simulink model "case3"  (R2024b)
settings: Solver=FixedStepAuto  StartTime=0  StopTime=1  FixedStep=1e-7  RelTol=1e-3
values from neighbouring files (symbols this model uses):
  SG_D_1_D = 0.01056    [IEEE9_case_parameters.m]    (also in case1_parameters.m; case2_parameters.m; case3_parameters.m; case4_parameters.m)
  SG_D_1_EnableSaturation = 0    [IEEE9_case_parameters.m]    (also in case1_parameters.m; case2_parameters.m; case3_parameters.m; case4_parameters.m)
  SG_D_1_f0 = 60    [IEEE9_case_parameters.m]    (also in case1_parameters.m; case2_parameters.m; case3_parameters.m; case4_parameters.m)
  SG_D_1_H = 7.5    [IEEE9_case_parameters.m]    (also in case1_parameters.m; case2_parameters.m; case3_parameters.m; case4_parameters.m)
  SG_D_1_K_A = 20    [IEEE9_case_parameters.m]    (also in case1_parameters.m; case2_parameters.m; case3_parameters.m; case4_parameters.m)
  SG_D_1_K_E = 1.000000e+1    (= 10)    [IEEE9_case_parameters.m]    (also in case1_parameters.m; case2_parameters.m; case3_parameters.m; case4_parameters.m)
  SG_D_1_K_F = 2.363    [IEEE9_case_parameters.m]    (also in case1_parameters.m; case2_parameters.m; case3_parameters.m; case4_parameters.m)
  SG_D_1_K_s = 0.5    [IEEE9_case_parameters.m]    (also in case1_parameters.m = 5; case2_parameters.m = 5; case3_parameters.m = 5; case4_parameters.m = 5)
  SG_D_1_R_a = 0.001088    [IEEE9_case_parameters.m]    (also in case1_parameters.m; case2_parameters.m; case3_parameters.m; case4_parameters.m)
  SG_D_1_S_A = 1    [IEEE9_case_parameters.m]    (also in case1_parameters.m; case2_parameters.m; case3_parameters.m; case4_parameters.m)
  SG_D_1_S_B = 0.103    [IEEE9_case_parameters.m]    (also in case1_parameters.m; case2_parameters.m; case3_parameters.m; case4_parameters.m)
  SG_D_1_S_N = 10.659857    [IEEE9_case_parameters.m]    (also in case1_parameters.m; case2_parameters.m; case3_parameters.m; case4_parameters.m)
  SG_D_1_SpeedPara = 200    [IEEE9_case_parameters.m]    (also in case1_parameters.m; case2_parameters.m; case3_parameters.m; case4_parameters.m)
  SG_D_1_T_0 = 0.720173    [IEEE9_case_parameters.m]    (also in case1_parameters.m = 0.755522; case2_parameters.m = 0.808931; case3_parameters.m = 0.869402; case4_parameters.m = 0.729316)
  SG_D_1_T_1 = 0.3    [IEEE9_case_parameters.m]    (also in case1_parameters.m; case2_parameters.m; case3_parameters.m; case4_parameters.m)
  SG_D_1_T_2 = 0.05    [IEEE9_case_parameters.m]    (also in case1_parameters.m; case2_parameters.m; case3_parameters.m; case4_parameters.m)
  SG_D_1_T_3 = 0.02    [IEEE9_case_parameters.m]    (also in case1_parameters.m; case2_parameters.m; case3_parameters.m; case4_parameters.m)
  SG_D_1_T_4 = 0.005    [IEEE9_case_parameters.m]    (also in case1_parameters.m; case2_parameters.m; case3_parameters.m; case4_parameters.m)
  SG_D_1_T_A = 0.02    [IEEE9_case_parameters.m]    (also in case1_parameters.m; case2_parameters.m; case3_parameters.m; case4_parameters.m)
  SG_D_1_T_dd = 8.000000e+0    (= 8)    [IEEE9_case_parameters.m]    (also in case1_parameters.m; case2_parameters.m; case3_parameters.m; case4_parameters.m)
  SG_D_1_T_ddd = 0.04    [IEEE9_case_parameters.m]    (also in case1_parameters.m; case2_parameters.m; case3_parameters.m; case4_parameters.m)
  SG_D_1_T_E = 0.314    [IEEE9_case_parameters.m]    (also in case1_parameters.m; case2_parameters.m; case3_parameters.m; case4_parameters.m)
  SG_D_1_T_F = 0.35    [IEEE9_case_parameters.m]    (also in case1_parameters.m; case2_parameters.m; case3_parameters.m; case4_parameters.m)
  SG_D_1_T_qd = 0.8    [IEEE9_case_parameters.m]    (also in case1_parameters.m; case2_parameters.m; case3_parameters.m; case4_parameters.m)
  SG_D_1_T_qdd = 0.02    [IEEE9_case_parameters.m]    (also in case1_parameters.m; case2_parameters.m; case3_parameters.m; case4_parameters.m)
  SG_D_1_T_speed = 0.1    [IEEE9_case_parameters.m]    (also in case1_parameters.m = 200; case2_parameters.m = 200; case3_parameters.m = 200; case4_parameters.m = 200)
  SG_D_1_T_w = 0.5    [IEEE9_case_parameters.m]    (also in case1_parameters.m; case2_parameters.m; case3_parameters.m; case4_parameters.m)
  SG_D_1_V_ref = 1.990276    [IEEE9_case_parameters.m]    (also in case1_parameters.m = 2.042296; case2_parameters.m = 2.051388; case3_parameters.m = 2.089584; case4_parameters.m = 2.01845)
  SG_D_1_w_ref = 376.991118    [IEEE9_case_parameters.m]    (also in case1_parameters.m; case2_parameters.m; case3_parameters.m; case4_parameters.m)
  SG_D_1_wb = 6.000000e+1    (= 60)    [IEEE9_case_parameters.m]    (also in case1_parameters.m; case2_parameters.m; case3_parameters.m; case4_parameters.m)
  SG_D_1_x_d = 1.9    [IEEE9_case_parameters.m]    (also in case1_parameters.m; case2_parameters.m; case3_parameters.m; case4_parameters.m)
  SG_D_1_x_dd = 0.302    [IEEE9_case_parameters.m]    (also in case1_parameters.m; case2_parameters.m; case3_parameters.m; case4_parameters.m)
  SG_D_1_x_ddd = 0.204    [IEEE9_case_parameters.m]    (also in case1_parameters.m; case2_parameters.m; case3_parameters.m; case4_parameters.m)
  SG_D_1_x_l = 0.05    [IEEE9_case_parameters.m]    (also in case1_parameters.m; case2_parameters.m; case3_parameters.m; case4_parameters.m)
  SG_D_1_x_q = 1.3    [IEEE9_case_parameters.m]    (also in case1_parameters.m; case2_parameters.m; case3_parameters.m; case4_parameters.m)
  SG_D_1_x_qd = 0.5    [IEEE9_case_parameters.m]    (also in case1_parameters.m; case2_parameters.m; case3_parameters.m; case4_parameters.m)
  SG_D_1_x_qdd = 0.3    [IEEE9_case_parameters.m]    (also in case1_parameters.m; case2_parameters.m; case3_parameters.m; case4_parameters.m)
  SG_D_2_D = 0.02    [IEEE9_case_parameters.m]    (also in case1_parameters.m; case2_parameters.m; case3_parameters.m; case4_parameters.m)
  SG_D_2_EnableSaturation = 0    [IEEE9_case_parameters.m]    (also in case1_parameters.m; case2_parameters.m; case3_parameters.m; case4_parameters.m)
  SG_D_2_f0 = 60    [IEEE9_case_parameters.m]    (also in case1_parameters.m; case2_parameters.m; case3_parameters.m; case4_parameters.m)
  SG_D_2_H = 8.000000e+0    (= 8)    [IEEE9_case_parameters.m]    (also in case1_parameters.m; case2_parameters.m; case3_parameters.m; case4_parameters.m)
  SG_D_2_K_A = 20    [IEEE9_case_parameters.m]    (also in case1_parameters.m; case2_parameters.m; case3_parameters.m; case4_parameters.m)
  SG_D_2_K_E = 1.000000e+1    (= 10)    [IEEE9_case_parameters.m]    (also in case1_parameters.m; case2_parameters.m; case3_parameters.m; case4_parameters.m)
  SG_D_2_K_F = 2.363    [IEEE9_case_parameters.m]    (also in case1_parameters.m; case2_parameters.m; case3_parameters.m; case4_parameters.m)
  SG_D_2_K_s = 0.5    [IEEE9_case_parameters.m]    (also in case1_parameters.m = 4; case2_parameters.m = 4; case3_parameters.m = 4; case4_parameters.m = 4)
  SG_D_2_R_a = 0.001088    [IEEE9_case_parameters.m]    (also in case1_parameters.m; case2_parameters.m; case3_parameters.m; case4_parameters.m)
  SG_D_2_S_A = 1    [IEEE9_case_parameters.m]    (also in case1_parameters.m; case2_parameters.m; case3_parameters.m; case4_parameters.m)
  SG_D_2_S_B = 0.103    [IEEE9_case_parameters.m]    (also in case1_parameters.m; case2_parameters.m; case3_parameters.m; case4_parameters.m)
  SG_D_2_S_N = 10.659857    [IEEE9_case_parameters.m]    (also in case1_parameters.m; case2_parameters.m; case3_parameters.m; case4_parameters.m)
  SG_D_2_SpeedPara = 200    [IEEE9_case_parameters.m]    (also in case1_parameters.m; case2_parameters.m; case3_parameters.m; case4_parameters.m)
  SG_D_2_T_0 = 1.632913    [IEEE9_case_parameters.m]    (also in case1_parameters.m = 1.632925; case2_parameters.m = 1.632915; case3_parameters.m = 1.632914; case4_parameters.m = 1.632927)
  SG_D_2_T_1 = 0.2    [IEEE9_case_parameters.m]    (also in case1_parameters.m; case2_parameters.m; case3_parameters.m; case4_parameters.m)
  SG_D_2_T_2 = 0.05    [IEEE9_case_parameters.m]    (also in case1_parameters.m; case2_parameters.m; case3_parameters.m; case4_parameters.m)
  SG_D_2_T_3 = 0.02    [IEEE9_case_parameters.m]    (also in case1_parameters.m; case2_parameters.m; case3_parameters.m; case4_parameters.m)
  SG_D_2_T_4 = 0.005    [IEEE9_case_parameters.m]    (also in case1_parameters.m; case2_parameters.m; case3_parameters.m; case4_parameters.m)
  SG_D_2_T_A = 0.02    [IEEE9_case_parameters.m]    (also in case1_parameters.m; case2_parameters.m; case3_parameters.m; case4_parameters.m)
  SG_D_2_T_dd = 7.9    [IEEE9_case_parameters.m]    (also in case1_parameters.m; case2_parameters.m; case3_parameters.m; case4_parameters.m)
  SG_D_2_T_ddd = 0.04    [IEEE9_case_parameters.m]    (also in case1_parameters.m; case2_parameters.m; case3_parameters.m; case4_parameters.m)
  SG_D_2_T_E = 0.314    [IEEE9_case_parameters.m]    (also in case1_parameters.m; case2_parameters.m; case3_parameters.m; case4_parameters.m)
  SG_D_2_T_F = 0.35    [IEEE9_case_parameters.m]    (also in case1_parameters.m; case2_parameters.m; case3_parameters.m; case4_parameters.m)
  SG_D_2_T_qd = 0.8    [IEEE9_case_parameters.m]    (also in case1_parameters.m; case2_parameters.m; case3_parameters.m; case4_parameters.m)
  SG_D_2_T_qdd = 0.015    [IEEE9_case_parameters.m]    (also in case1_parameters.m; case2_parameters.m; case3_parameters.m; case4_parameters.m)
  SG_D_2_T_speed = 0.1    [IEEE9_case_parameters.m]    (also in case1_parameters.m = 150; case2_parameters.m = 150; case3_parameters.m = 150; case4_parameters.m = 150)
  SG_D_2_T_w = 0.35    [IEEE9_case_parameters.m]    (also in case1_parameters.m; case2_parameters.m; case3_parameters.m; case4_parameters.m)
  SG_D_2_V_ref = 2.58547    [IEEE9_case_parameters.m]    (also in case1_parameters.m = 2.597896; case2_parameters.m = 2.587136; case3_parameters.m = 2.586042; case4_parameters.m = 2.599679)
  SG_D_2_w_ref = 376.991118    [IEEE9_case_parameters.m]    (also in case1_parameters.m; case2_parameters.m; case3_parameters.m; case4_parameters.m)
  SG_D_2_wb = 6.000000e+1    (= 60)    [IEEE9_case_parameters.m]    (also in case1_parameters.m; case2_parameters.m; case3_parameters.m; case4_parameters.m)
  SG_D_2_x_d = 1.8    [IEEE9_case_parameters.m]    (also in case1_parameters.m; case2_parameters.m; case3_parameters.m; case4_parameters.m)
  SG_D_2_x_dd = 0.302    [IEEE9_case_parameters.m]    (also in case1_parameters.m; case2_parameters.m; case3_parameters.m; case4_parameters.m)
  SG_D_2_x_ddd = 0.204    [IEEE9_case_parameters.m]    (also in case1_parameters.m; case2_parameters.m; case3_parameters.m; case4_parameters.m)
  SG_D_2_x_l = 0.05    [IEEE9_case_parameters.m]    (also in case1_parameters.m; case2_parameters.m; case3_parameters.m; case4_parameters.m)
  SG_D_2_x_q = 1.25    [IEEE9_case_parameters.m]    (also in case1_parameters.m; case2_parameters.m; case3_parameters.m; case4_parameters.m)
  SG_D_2_x_qd = 0.5    [IEEE9_case_parameters.m]    (also in case1_parameters.m; case2_parameters.m; case3_parameters.m; case4_parameters.m)
  SG_D_2_x_qdd = 0.3    [IEEE9_case_parameters.m]    (also in case1_parameters.m; case2_parameters.m; case3_parameters.m; case4_parameters.m)
  SG_D_3_D = 0.02    [IEEE9_case_parameters.m]    (also in case1_parameters.m; case2_parameters.m; case3_parameters.m; case4_parameters.m)
  SG_D_3_EnableSaturation = 0    [IEEE9_case_parameters.m]    (also in case1_parameters.m; case2_parameters.m; case3_parameters.m; case4_parameters.m)
  SG_D_3_f0 = 60    [IEEE9_case_parameters.m]    (also in case1_parameters.m; case2_parameters.m; case3_parameters.m; case4_parameters.m)
  SG_D_3_H = 7.7    [IEEE9_case_parameters.m]    (also in case1_parameters.m; case2_parameters.m; case3_parameters.m; case4_parameters.m)
  SG_D_3_K_A = 20    [IEEE9_case_parameters.m]    (also in case1_parameters.m; case2_parameters.m; case3_parameters.m; case4_parameters.m)
  SG_D_3_K_E = 1.000000e+1    (= 10)    [IEEE9_case_parameters.m]    (also in case1_parameters.m; case2_parameters.m; case3_parameters.m; case4_parameters.m)
  SG_D_3_K_F = 2.363    [IEEE9_case_parameters.m]    (also in case1_parameters.m; case2_parameters.m; case3_parameters.m; case4_parameters.m)
  SG_D_3_K_s = 0.2    [IEEE9_case_parameters.m]    (also in case1_parameters.m = 2; case2_parameters.m = 2; case3_parameters.m = 2; case4_parameters.m = 2)
  SG_D_3_R_a = 0.001088    [IEEE9_case_parameters.m]    (also in case1_parameters.m; case2_parameters.m; case3_parameters.m; case4_parameters.m)
  SG_D_3_S_A = 1    [IEEE9_case_parameters.m]    (also in case1_parameters.m; case2_parameters.m; case3_parameters.m; case4_parameters.m)
  SG_D_3_S_B = 0.103    [IEEE9_case_parameters.m]    (also in case1_parameters.m; case2_parameters.m; case3_parameters.m; case4_parameters.m)
  SG_D_3_S_N = 10.659857    [IEEE9_case_parameters.m]    (also in case1_parameters.m; case2_parameters.m; case3_parameters.m; case4_parameters.m)
  SG_D_3_SpeedPara = 200    [IEEE9_case_parameters.m]    (also in case1_parameters.m; case2_parameters.m; case3_parameters.m; case4_parameters.m)
  SG_D_3_T_0 = 0.850788    [IEEE9_case_parameters.m]    (also in case1_parameters.m = 0.850786; case2_parameters.m = 0.850787; case3_parameters.m; case4_parameters.m = 0.850786)
  SG_D_3_T_1 = 0.2    [IEEE9_case_parameters.m]    (also in case1_parameters.m; case2_parameters.m; case3_parameters.m; case4_parameters.m)
  SG_D_3_T_2 = 0.05    [IEEE9_case_parameters.m]    (also in case1_parameters.m; case2_parameters.m; case3_parameters.m; case4_parameters.m)
  SG_D_3_T_3 = 0.02    [IEEE9_case_parameters.m]    (also in case1_parameters.m; case2_parameters.m; case3_parameters.m; case4_parameters.m)
  SG_D_3_T_4 = 0.005    [IEEE9_case_parameters.m]    (also in case1_parameters.m; case2_parameters.m; case3_parameters.m; case4_parameters.m)
  SG_D_3_T_A = 0.02    [IEEE9_case_parameters.m]    (also in case1_parameters.m; case2_parameters.m; case3_parameters.m; case4_parameters.m)
  SG_D_3_T_dd = 8.1    [IEEE9_case_parameters.m]    (also in case1_parameters.m; case2_parameters.m; case3_parameters.m; case4_parameters.m)
  SG_D_3_T_ddd = 0.04    [IEEE9_case_parameters.m]    (also in case1_parameters.m; case2_parameters.m; case3_parameters.m; case4_parameters.m)
  SG_D_3_T_E = 0.314    [IEEE9_case_parameters.m]    (also in case1_parameters.m; case2_parameters.m; case3_parameters.m; case4_parameters.m)
  SG_D_3_T_F = 0.35    [IEEE9_case_parameters.m]    (also in case1_parameters.m; case2_parameters.m; case3_parameters.m; case4_parameters.m)
  SG_D_3_T_qd = 0.8    [IEEE9_case_parameters.m]    (also in case1_parameters.m; case2_parameters.m; case3_parameters.m; case4_parameters.m)
  SG_D_3_T_qdd = 0.015    [IEEE9_case_parameters.m]    (also in case1_parameters.m; case2_parameters.m; case3_parameters.m; case4_parameters.m)
  SG_D_3_T_speed = 0.1    [IEEE9_case_parameters.m]    (also in case1_parameters.m = 180; case2_parameters.m = 180; case3_parameters.m = 180; case4_parameters.m = 180)
  SG_D_3_T_w = 0.4    [IEEE9_case_parameters.m]    (also in case1_parameters.m; case2_parameters.m; case3_parameters.m; case4_parameters.m)
  SG_D_3_V_ref = 1.892727    [IEEE9_case_parameters.m]    (also in case1_parameters.m = 1.906439; case2_parameters.m = 1.895535; case3_parameters.m = 1.892105; case4_parameters.m = 1.906598)
  SG_D_3_w_ref = 376.991118    [IEEE9_case_parameters.m]    (also in case1_parameters.m; case2_parameters.m; case3_parameters.m; case4_parameters.m)
  SG_D_3_wb = 6.000000e+1    (= 60)    [IEEE9_case_parameters.m]    (also in case1_parameters.m; case2_parameters.m; case3_parameters.m; case4_parameters.m)
  SG_D_3_x_d = 1.85    [IEEE9_case_parameters.m]    (also in case1_parameters.m; case2_parameters.m; case3_parameters.m; case4_parameters.m)
  SG_D_3_x_dd = 0.302    [IEEE9_case_parameters.m]    (also in case1_parameters.m; case2_parameters.m; case3_parameters.m; case4_parameters.m)
  SG_D_3_x_ddd = 0.204    [IEEE9_case_parameters.m]    (also in case1_parameters.m; case2_parameters.m; case3_parameters.m; case4_parameters.m)
  SG_D_3_x_l = 0.05    [IEEE9_case_parameters.m]    (also in case1_parameters.m; case2_parameters.m; case3_parameters.m; case4_parameters.m)
  SG_D_3_x_q = 1.2    [IEEE9_case_parameters.m]    (also in case1_parameters.m; case2_parameters.m; case3_parameters.m; case4_parameters.m)
  SG_D_3_x_qd = 0.5    [IEEE9_case_parameters.m]    (also in case1_parameters.m; case2_parameters.m; case3_parameters.m; case4_parameters.m)
  SG_D_3_x_qdd = 0.3    [IEEE9_case_parameters.m]    (also in case1_parameters.m; case2_parameters.m; case3_parameters.m; case4_parameters.m)
(part 3 of 12)

== system case3/AC_1/d_id_load_7_block ==
  note: d_id_load_7 in case3
      | $376.991118430775\,\mathrm{iq}_{\mathrm{load},7}-1170.79515987921\,\mathrm{id}_{\mathrm{load},7}+1393.05476336183\,\mathrm{vd}_{\mathrm{bus},7}$
      | Automatically generated on 2025-10-31 19:02:10 .
  State_id_load_7_e043e : Inport
  State_iq_load_7_eee0e : Inport  Port=2
  State_vd_bus_7_6ab08 : Inport  Port=3
  Add_4a00a : Sum
  Add_ce181 : Sum
  Constant_-1170.79515987921_d27c0 : Constant  Value=-1170.79515987921
  Constant_1393.05476336183_3ce3e : Constant  Value=1393.05476336183
  Constant_376.991118430775_c116b : Constant  Value=376.991118430775
  Product_17dc1 : Product
  Product_565ff : Product
  Product_e7cd3 : Product
  Blockout_d_id_load_7_3ef5e : Outport
  wires:
  Constant_-1170.79515987921_d27c0/1 -> Product_17dc1/1
  Product_565ff/1 -> Add_4a00a/2
  State_id_load_7_e043e/1 -> Product_17dc1/2
  Constant_376.991118430775_c116b/1 -> Product_565ff/1
  Product_17dc1/1 -> Add_4a00a/1
  State_iq_load_7_eee0e/1 -> Product_565ff/2
  Constant_1393.05476336183_3ce3e/1 -> Product_e7cd3/1
  State_vd_bus_7_6ab08/1 -> Product_e7cd3/2
  Add_4a00a/1 -> Add_ce181/1
  Product_e7cd3/1 -> Add_ce181/2
  Add_ce181/1 -> Blockout_d_id_load_7_3ef5e/1

== system case3/AC_1/d_id_load_9_block ==
  note: d_id_load_9 in case3
      | $376.991118430775\,\mathrm{iq}_{\mathrm{load},9}-1024.44576485514\,\mathrm{id}_{\mathrm{load},9}+1663.3851206221\,\mathrm{vd}_{\mathrm{bus},9}$
      | Automatically generated on 2025-10-31 19:02:12 .
  State_id_load_9_00ea3 : Inport
  State_iq_load_9_29708 : Inport  Port=2
  State_vd_bus_9_36e95 : Inport  Port=3
  Add_12a09 : Sum
  Add_395e0 : Sum
  Constant_-1024.44576485514_f0212 : Constant  Value=-1024.44576485514
  Constant_1663.3851206221_94e84 : Constant  Value=1663.3851206221
  Constant_376.991118430775_61265 : Constant  Value=376.991118430775
  Product_55f5f : Product
  Product_af126 : Product
  Product_c42b8 : Product
  Blockout_d_id_load_9_781d1 : Outport
  wires:
  Constant_-1024.44576485514_f0212/1 -> Product_55f5f/1
  Product_af126/1 -> Add_12a09/2
  State_id_load_9_00ea3/1 -> Product_55f5f/2
  Constant_376.991118430775_61265/1 -> Product_af126/1
  Product_55f5f/1 -> Add_12a09/1
  State_iq_load_9_29708/1 -> Product_af126/2
  Constant_1663.3851206221_94e84/1 -> Product_c42b8/1
  State_vd_bus_9_36e95/1 -> Product_c42b8/2
  Add_12a09/1 -> Add_395e0/1
  Product_c42b8/1 -> Add_395e0/2
  Add_395e0/1 -> Blockout_d_id_load_9_781d1/1

== system case3/AC_1/d_iq_line_1_4_block ==
  note: d_iq_line_1_4 in case3
      | $6255.26744708076\,\mathrm{vq}_{\mathrm{bus},1}-376.991118430775\,\mathrm{id}_{\mathrm{line},1,4}-6255.26744708076\,\mathrm{vq}_{\mathrm{bus},4}$
      | Automatically generated on 2025-10-31 19:02:16 .
  State_id_line_1_4_1c233 : Inport
  State_vq_bus_1_eaf9d : Inport  Port=2
  State_vq_bus_4_44892 : Inport  Port=3
  Add_1d419 : Sum
  Constant_-376.991118430775_cdd09 : Constant  Value=-376.991118430775
  Constant_6255.26744708076_966f6 : Constant  Value=6255.26744708076
  Constant_6255.26744708076_c9a13 : Constant  Value=6255.26744708076
  Product_48e5f : Product
  Product_99397 : Product
  Product_c5425 : Product
  Subtract_80c11 : Sum  Inputs=+-
  Blockout_d_iq_line_1_4_64f6a : Outport
  wires:
  Constant_-376.991118430775_cdd09/1 -> Product_c5425/1
  Product_99397/1 -> Add_1d419/2
  State_id_line_1_4_1c233/1 -> Product_c5425/2
  Constant_6255.26744708076_966f6/1 -> Product_99397/1
  Product_c5425/1 -> Add_1d419/1
  Subtract_80c11/1 -> Blockout_d_iq_line_1_4_64f6a/1
  State_vq_bus_1_eaf9d/1 -> Product_99397/2
  Constant_6255.26744708076_c9a13/1 -> Product_48e5f/1
  State_vq_bus_4_44892/1 -> Product_48e5f/2
  Add_1d419/1 -> Subtract_80c11/1
  Product_48e5f/1 -> Subtract_80c11/2

== system case3/AC_1/d_iq_line_3_6_block ==
  note: d_iq_line_3_6 in case3
      | $6148.52226880293\,\mathrm{vq}_{\mathrm{bus},3}-376.991118430775\,\mathrm{id}_{\mathrm{line},3,6}-6148.52226880293\,\mathrm{vq}_{\mathrm{bus},6}$
      | Automatically generated on 2025-10-31 19:02:23 .
  State_id_line_3_6_f6ca7 : Inport
  State_vq_bus_3_2a06c : Inport  Port=2
  State_vq_bus_6_a5f6f : Inport  Port=3
  Add_32586 : Sum
  Constant_-376.991118430775_110a1 : Constant  Value=-376.991118430775
  Constant_6148.52226880293_1ad39 : Constant  Value=6148.52226880293
  Constant_6148.52226880293_30567 : Constant  Value=6148.52226880293
  Product_6139a : Product
  Product_c1ce3 : Product
  Product_c8059 : Product
  Subtract_d1a7b : Sum  Inputs=+-
  Blockout_d_iq_line_3_6_89a9d : Outport
  wires:
  Constant_-376.991118430775_110a1/1 -> Product_6139a/1
  Product_c1ce3/1 -> Add_32586/2
  State_id_line_3_6_f6ca7/1 -> Product_6139a/2
  Constant_6148.52226880293_1ad39/1 -> Product_c1ce3/1
  Product_6139a/1 -> Add_32586/1
  State_vq_bus_3_2a06c/1 -> Product_c1ce3/2
  Constant_6148.52226880293_30567/1 -> Product_c8059/1
  State_vq_bus_6_a5f6f/1 -> Product_c8059/2
  Add_32586/1 -> Subtract_d1a7b/1
  Product_c8059/1 -> Subtract_d1a7b/2
  Subtract_d1a7b/1 -> Blockout_d_iq_line_3_6_89a9d/1

== system case3/AC_1/d_iq_line_4_5_block ==
  note: d_iq_line_4_5 in case3
      | $3916.3413581723\,\mathrm{vq}_{\mathrm{bus},4}-71.2470020354664\,\mathrm{iq}_{\mathrm{line},4,5}-376.991118430775\,\mathrm{id}_{\mathrm{line},4,5}-3916.3413581723\,\mathrm{vq}_{\mathrm{bus},5}$
      | Automatically generated on 2025-10-31 19:02:18 .
  State_id_line_4_5_24b18 : Inport
  State_iq_line_4_5_05a1c : Inport  Port=2
  State_vq_bus_4_3c986 : Inport  Port=3
  State_vq_bus_5_9ee14 : Inport  Port=4
  Add_55fd1 : Sum
  Constant_-376.991118430775_25c53 : Constant  Value=-376.991118430775
  Constant_3916.3413581723_02aa0 : Constant  Value=3916.3413581723
  Constant_3916.3413581723_e3111 : Constant  Value=3916.3413581723
  Constant_71.2470020354664_483c4 : Constant  Value=71.2470020354664
  Product_6d1c1 : Product
  Product_d744e : Product
  Product_de414 : Product
  Product_e84cd : Product
  Subtract_8c007 : Sum  Inputs=+-
  Subtract_dfdcb : Sum  Inputs=+-
  Blockout_d_iq_line_4_5_2a670 : Outport
  wires:
  Constant_-376.991118430775_25c53/1 -> Product_6d1c1/1
  Constant_71.2470020354664_483c4/1 -> Product_d744e/1
  State_id_line_4_5_24b18/1 -> Product_6d1c1/2
  State_iq_line_4_5_05a1c/1 -> Product_d744e/2
  Product_6d1c1/1 -> Subtract_dfdcb/1
  Constant_3916.3413581723_02aa0/1 -> Product_e84cd/1
  Product_d744e/1 -> Subtract_dfdcb/2
  State_vq_bus_4_3c986/1 -> Product_e84cd/2
  Subtract_dfdcb/1 -> Add_55fd1/1
  Product_e84cd/1 -> Add_55fd1/2
  Constant_3916.3413581723_e3111/1 -> Product_de414/1
  State_vq_bus_5_9ee14/1 -> Product_de414/2
  Add_55fd1/1 -> Subtract_8c007/1
  Product_de414/1 -> Subtract_8c007/2
  Subtract_8c007/1 -> Blockout_d_iq_line_4_5_2a670/1

== system case3/AC_1/d_iq_line_5_6_block ==
  note: d_iq_line_5_6 in case3
      | $2119.43179383442\,\mathrm{vq}_{\mathrm{bus},5}-88.4547554682538\,\mathrm{iq}_{\mathrm{line},5,6}-376.991118430775\,\mathrm{id}_{\mathrm{line},5,6}-2119.43179383442\,\mathrm{vq}_{\mathrm{bus},6}$
      | Automatically generated on 2025-10-31 19:02:21 .
  State_id_line_5_6_f3a7a : Inport
  State_iq_line_5_6_affd3 : Inport  Port=2
  State_vq_bus_5_6825f : Inport  Port=3
  State_vq_bus_6_7d333 : Inport  Port=4
  Add_b4ad5 : Sum
  Constant_-376.991118430775_4a976 : Constant  Value=-376.991118430775
  Constant_2119.43179383442_0d754 : Constant  Value=2119.43179383442
  Constant_2119.43179383442_108e5 : Constant  Value=2119.43179383442
  Constant_88.4547554682538_e4ce4 : Constant  Value=88.4547554682538
  Product_06499 : Product
  Product_0dc6d : Product
  Product_761ae : Product
  Product_eeb40 : Product
  Subtract_8af08 : Sum  Inputs=+-
  Subtract_c0488 : Sum  Inputs=+-
  Blockout_d_iq_line_5_6_beac2 : Outport
  wires:
  Constant_-376.991118430775_4a976/1 -> Product_761ae/1
  Constant_88.4547554682538_e4ce4/1 -> Product_0dc6d/1
  Subtract_8af08/1 -> Blockout_d_iq_line_5_6_beac2/1
  State_id_line_5_6_f3a7a/1 -> Product_761ae/2
  State_iq_line_5_6_affd3/1 -> Product_0dc6d/2
  Product_761ae/1 -> Subtract_c0488/1
  Constant_2119.43179383442_0d754/1 -> Product_06499/1
  Product_0dc6d/1 -> Subtract_c0488/2
  Product_eeb40/1 -> Subtract_8af08/2
  State_vq_bus_5_6825f/1 -> Product_06499/2
  Subtract_c0488/1 -> Add_b4ad5/1
  Product_06499/1 -> Add_b4ad5/2
  Constant_2119.43179383442_108e5/1 -> Product_eeb40/1
  State_vq_bus_6_7d333/1 -> Product_eeb40/2
  Add_b4ad5/1 -> Subtract_8af08/1

== system case3/AC_1/d_iq_line_6_7_block ==
  note: d_iq_line_6_7 in case3
      | $3574.43854118901\,\mathrm{vq}_{\mathrm{bus},6}-45.5189179671035\,\mathrm{iq}_{\mathrm{line},6,7}-376.991118430775\,\mathrm{id}_{\mathrm{line},6,7}-3574.43854118901\,\mathrm{vq}_{\mathrm{bus},7}$
      | Automatically generated on 2025-10-31 19:02:26 .
  State_id_line_6_7_cd5da : Inport
  State_iq_line_6_7_f3824 : Inport  Port=2
  State_vq_bus_6_01e40 : Inport  Port=3
  State_vq_bus_7_d9bfc : Inport  Port=4
  Add_3e19f : Sum
  Constant_-376.991118430775_ca8cb : Constant  Value=-376.991118430775
  Constant_3574.43854118901_6a426 : Constant  Value=3574.43854118901
  Constant_3574.43854118901_6d105 : Constant  Value=3574.43854118901
  Constant_45.5189179671035_112d0 : Constant  Value=45.5189179671035
  Product_8fb0e : Product
  Product_a3e25 : Product
  Product_c7267 : Product
  Product_efecf : Product
  Subtract_6615b : Sum  Inputs=+-
  Subtract_a965d : Sum  Inputs=+-
  Blockout_d_iq_line_6_7_3df17 : Outport
  wires:
  Constant_-376.991118430775_ca8cb/1 -> Product_8fb0e/1
  Constant_45.5189179671035_112d0/1 -> Product_a3e25/1
  State_id_line_6_7_cd5da/1 -> Product_8fb0e/2
  State_iq_line_6_7_f3824/1 -> Product_a3e25/2
  Product_8fb0e/1 -> Subtract_a965d/1
  Constant_3574.43854118901_6d105/1 -> Product_efecf/1
  Product_a3e25/1 -> Subtract_a965d/2
  State_vq_bus_6_01e40/1 -> Product_efecf/2
  Subtract_a965d/1 -> Add_3e19f/1
  Product_efecf/1 -> Add_3e19f/2
  Constant_3574.43854118901_6a426/1 -> Product_c7267/1
  State_vq_bus_7_d9bfc/1 -> Product_c7267/2
  Add_3e19f/1 -> Subtract_6615b/1
  Product_c7267/1 -> Subtract_6615b/2
  Subtract_6615b/1 -> Blockout_d_iq_line_6_7_3df17/1

== system case3/AC_1/d_iq_line_7_8_block ==
  note: d_iq_line_7_8 in case3
      | $5004.21395766461\,\mathrm{vq}_{\mathrm{bus},7}-45.5189179671035\,\mathrm{iq}_{\mathrm{line},7,8}-376.991118430775\,\mathrm{id}_{\mathrm{line},7,8}-5004.21395766461\,\mathrm{vq}_{\mathrm{bus},8}$
      | Automatically generated on 2025-10-31 19:02:28 .
  State_id_line_7_8_b4d16 : Inport
  State_iq_line_7_8_0ca45 : Inport  Port=2
  State_vq_bus_7_50286 : Inport  Port=3
  State_vq_bus_8_3d863 : Inport  Port=4
  Add_1c111 : Sum
  Constant_-376.991118430775_be40d : Constant  Value=-376.991118430775
  Constant_45.5189179671035_a41f8 : Constant  Value=45.5189179671035
  Constant_5004.21395766461_8dc94 : Constant  Value=5004.21395766461
  Constant_5004.21395766461_aa5bd : Constant  Value=5004.21395766461
  Product_4bb88 : Product
  Product_7847e : Product
  Product_c0882 : Product
  Product_f5c9c : Product
  Subtract_4028b : Sum  Inputs=+-
  Subtract_e4f7a : Sum  Inputs=+-
  Blockout_d_iq_line_7_8_5ff90 : Outport
  wires:
  Constant_-376.991118430775_be40d/1 -> Product_f5c9c/1
  Constant_45.5189179671035_a41f8/1 -> Product_c0882/1
  State_id_line_7_8_b4d16/1 -> Product_f5c9c/2
  State_iq_line_7_8_0ca45/1 -> Product_c0882/2
  Product_f5c9c/1 -> Subtract_4028b/1
  Constant_5004.21395766461_8dc94/1 -> Product_4bb88/1
  Product_c0882/1 -> Subtract_4028b/2
  State_vq_bus_7_50286/1 -> Product_4bb88/2
  Subtract_4028b/1 -> Add_1c111/1
  Product_4bb88/1 -> Add_1c111/2
  Constant_5004.21395766461_aa5bd/1 -> Product_7847e/1
  State_vq_bus_8_3d863/1 -> Product_7847e/2
  Add_1c111/1 -> Subtract_e4f7a/1
  Product_7847e/1 -> Subtract_e4f7a/2
  Subtract_e4f7a/1 -> Blockout_d_iq_line_7_8_5ff90/1

== system case3/AC_1/d_iq_line_8_2_block ==
  note: d_iq_line_8_2 in case3
      | $5764.85447922963\,\mathrm{vq}_{\mathrm{bus},8}-5764.85447922963\,\mathrm{vq}_{\mathrm{bus},2}-376.991118430775\,\mathrm{id}_{\mathrm{line},8,2}$
      | Automatically generated on 2025-10-31 19:02:31 .
  State_id_line_8_2_73741 : Inport
  State_vq_bus_2_813db : Inport  Port=2
  State_vq_bus_8_3e61a : Inport  Port=3
  Add_ca283 : Sum
  Constant_-376.991118430775_fbd35 : Constant  Value=-376.991118430775
  Constant_5764.85447922963_0bcbf : Constant  Value=5764.85447922963
  Constant_5764.85447922963_c259e : Constant  Value=5764.85447922963
  Product_3857e : Product
  Product_3c608 : Product
  Product_68149 : Product
  Subtract_74c0a : Sum  Inputs=+-
  Blockout_d_iq_line_8_2_aa3d3 : Outport
  wires:
  Constant_-376.991118430775_fbd35/1 -> Product_68149/1
  Product_3c608/1 -> Subtract_74c0a/2
  State_id_line_8_2_73741/1 -> Product_68149/2
  Constant_5764.85447922963_c259e/1 -> Product_3c608/1
  Product_68149/1 -> Subtract_74c0a/1
  State_vq_bus_2_813db/1 -> Product_3c608/2
  Constant_5764.85447922963_0bcbf/1 -> Product_3857e/1
  State_vq_bus_8_3e61a/1 -> Product_3857e/2
  Subtract_74c0a/1 -> Add_ca283/1
  Product_3857e/1 -> Add_ca283/2
  Add_ca283/1 -> Blockout_d_iq_line_8_2_aa3d3/1

== system case3/AC_1/d_iq_line_8_9_block ==
  note: d_iq_line_8_9 in case3
      | $2237.90934752703\,\mathrm{vq}_{\mathrm{bus},8}-76.6354307608378\,\mathrm{iq}_{\mathrm{line},8,9}-376.991118430775\,\mathrm{id}_{\mathrm{line},8,9}-2237.90934752703\,\mathrm{vq}_{\mathrm{bus},9}$
      | Automatically generated on 2025-10-31 19:02:33 .
  State_id_line_8_9_642ba : Inport
  State_iq_line_8_9_96dc9 : Inport  Port=2
  State_vq_bus_8_011bb : Inport  Port=3
  State_vq_bus_9_8381b : Inport  Port=4
  Add_d3da0 : Sum
  Constant_-376.991118430775_f1810 : Constant  Value=-376.991118430775
  Constant_2237.90934752703_100b9 : Constant  Value=2237.90934752703
  Constant_2237.90934752703_bc38b : Constant  Value=2237.90934752703
  Constant_76.6354307608378_8c9a2 : Constant  Value=76.6354307608378
  Product_112b4 : Product
  Product_25dda : Product
  Product_38f36 : Product
  Product_c1704 : Product
  Subtract_3d788 : Sum  Inputs=+-
  Subtract_6f12d : Sum  Inputs=+-
  Blockout_d_iq_line_8_9_02383 : Outport
  wires:
  Constant_-376.991118430775_f1810/1 -> Product_25dda/1
  Constant_76.6354307608378_8c9a2/1 -> Product_c1704/1
  State_id_line_8_9_642ba/1 -> Product_25dda/2
  State_iq_line_8_9_96dc9/1 -> Product_c1704/2
  Product_25dda/1 -> Subtract_6f12d/1
  Constant_2237.90934752703_bc38b/1 -> Product_38f36/1
  Product_c1704/1 -> Subtract_6f12d/2
  State_vq_bus_8_011bb/1 -> Product_38f36/2
  Subtract_6f12d/1 -> Add_d3da0/1
  Product_38f36/1 -> Add_d3da0/2
  Constant_2237.90934752703_100b9/1 -> Product_112b4/1
  Add_d3da0/1 -> Subtract_3d788/1
  State_vq_bus_9_8381b/1 -> Product_112b4/2
  Product_112b4/1 -> Subtract_3d788/2
  Subtract_3d788/1 -> Blockout_d_iq_line_8_9_02383/1

== system case3/AC_1/d_iq_line_9_4_block ==
  note: d_iq_line_9_4 in case3
      | $4238.86358766884\,\mathrm{vq}_{\mathrm{bus},9}-45.3614130606429\,\mathrm{iq}_{\mathrm{line},9,4}-4238.86358766884\,\mathrm{vq}_{\mathrm{bus},4}-376.991118430775\,\mathrm{id}_{\mathrm{line},9,4}$
      | Automatically generated on 2025-10-31 19:02:36 .
  State_id_line_9_4_af562 : Inport
  State_iq_line_9_4_ffcdd : Inport  Port=2
  State_vq_bus_4_28404 : Inport  Port=3
  State_vq_bus_9_46860 : Inport  Port=4
  Add_2ee31 : Sum
  Constant_-376.991118430775_dd642 : Constant  Value=-376.991118430775
  Constant_4238.86358766884_116f6 : Constant  Value=4238.86358766884
  Constant_4238.86358766884_ffbde : Constant  Value=4238.86358766884
  Constant_45.3614130606429_7e441 : Constant  Value=45.3614130606429
  Product_0d4e3 : Product
  Product_37579 : Product
  Product_441f7 : Product
  Product_f12e6 : Product
  Subtract_a3b8f : Sum  Inputs=+-
  Subtract_debe8 : Sum  Inputs=+-
  Blockout_d_iq_line_9_4_72d66 : Outport
  wires:
  Constant_-376.991118430775_dd642/1 -> Product_441f7/1
  Constant_45.3614130606429_7e441/1 -> Product_0d4e3/1
  State_id_line_9_4_af562/1 -> Product_441f7/2
  State_iq_line_9_4_ffcdd/1 -> Product_0d4e3/2
  Product_441f7/1 -> Subtract_a3b8f/1
  Constant_4238.86358766884_116f6/1 -> Product_f12e6/1
  Product_0d4e3/1 -> Subtract_a3b8f/2
  State_vq_bus_4_28404/1 -> Product_f12e6/2
  Subtract_a3b8f/1 -> Subtract_debe8/1
  Product_f12e6/1 -> Subtract_debe8/2
  Constant_4238.86358766884_ffbde/1 -> Product_37579/1
  Add_2ee31/1 -> Blockout_d_iq_line_9_4_72d66/1
  State_vq_bus_9_46860/1 -> Product_37579/2
  Subtract_debe8/1 -> Add_2ee31/1
  Product_37579/1 -> Add_2ee31/2

== system case3/AC_1/d_iq_load_5_block ==
  note: d_iq_load_5 in case3
      | $1333.35238164348\,\mathrm{vq}_{\mathrm{bus},5}-1229.33491779484\,\mathrm{iq}_{\mathrm{load},5}-376.991118430775\,\mathrm{id}_{\mathrm{load},5}$
      | Automatically generated on 2025-10-31 19:02:09 .
  State_id_load_5_e1948 : Inport
  State_iq_load_5_68fca : Inport  Port=2
  State_vq_bus_5_03c1b : Inport  Port=3
  Add_2397b : Sum
  Constant_-376.991118430775_88d27 : Constant  Value=-376.991118430775
  Constant_1229.33491779484_3ec29 : Constant  Value=1229.33491779484
  Constant_1333.35238164348_d4a24 : Constant  Value=1333.35238164348
  Product_8108c : Product
  Product_b42b0 : Product
  Product_e05b1 : Product
  Subtract_211aa : Sum  Inputs=+-
  Blockout_d_iq_load_5_e65a1 : Outport
  wires:
  Constant_-376.991118430775_88d27/1 -> Product_b42b0/1
  Product_e05b1/1 -> Subtract_211aa/2
  State_id_load_5_e1948/1 -> Product_b42b0/2
  Constant_1229.33491779484_3ec29/1 -> Product_e05b1/1
  Product_b42b0/1 -> Subtract_211aa/1
  State_iq_load_5_68fca/1 -> Product_e05b1/2
  Constant_1333.35238164348_d4a24/1 -> Product_8108c/1
  State_vq_bus_5_03c1b/1 -> Product_8108c/2
  Subtract_211aa/1 -> Add_2397b/1
  Product_8108c/1 -> Add_2397b/2
  Add_2397b/1 -> Blockout_d_iq_load_5_e65a1/1

== system case3/AC_1/d_iq_load_7_block ==
  note: d_iq_load_7 in case3
      | $1393.05476336183\,\mathrm{vq}_{\mathrm{bus},7}-1170.79515987921\,\mathrm{iq}_{\mathrm{load},7}-376.991118430775\,\mathrm{id}_{\mathrm{load},7}$
      | Automatically generated on 2025-10-31 19:02:11 .
  State_id_load_7_f43ef : Inport
  State_iq_load_7_a1d5b : Inport  Port=2
  State_vq_bus_7_a3eff : Inport  Port=3
  Add_9694c : Sum
  Constant_-376.991118430775_645f4 : Constant  Value=-376.991118430775
  Constant_1170.79515987921_2311d : Constant  Value=1170.79515987921
  Constant_1393.05476336183_47307 : Constant  Value=1393.05476336183
  Product_3fdab : Product
  Product_e3269 : Product
  Product_f8db0 : Product
  Subtract_41138 : Sum  Inputs=+-
  Blockout_d_iq_load_7_43a8a : Outport
  wires:
  Constant_-376.991118430775_645f4/1 -> Product_3fdab/1
  Product_e3269/1 -> Subtract_41138/2
  State_id_load_7_f43ef/1 -> Product_3fdab/2
  Constant_1170.79515987921_2311d/1 -> Product_e3269/1
  Product_3fdab/1 -> Subtract_41138/1
  State_iq_load_7_a1d5b/1 -> Product_e3269/2
  Constant_1393.05476336183_47307/1 -> Product_f8db0/1
  State_vq_bus_7_a3eff/1 -> Product_f8db0/2
  Subtract_41138/1 -> Add_9694c/1
  Product_f8db0/1 -> Add_9694c/2
  Add_9694c/1 -> Blockout_d_iq_load_7_43a8a/1

== system case3/AC_1/d_iq_load_9_block ==
  note: d_iq_load_9 in case3
      | $1663.3851206221\,\mathrm{vq}_{\mathrm{bus},9}-1024.44576485514\,\mathrm{iq}_{\mathrm{load},9}-376.991118430775\,\mathrm{id}_{\mathrm{load},9}$
      | Automatically generated on 2025-10-31 19:02:13 .
  State_id_load_9_95b0f : Inport
  State_iq_load_9_9ab5c : Inport  Port=2
  State_vq_bus_9_4829d : Inport  Port=3
  Add_7623c : Sum
  Constant_-376.991118430775_ad088 : Constant  Value=-376.991118430775
  Constant_1024.44576485514_7c6f5 : Constant  Value=1024.44576485514
  Constant_1663.3851206221_38dd2 : Constant  Value=1663.3851206221
  Product_c5042 : Product
  Product_ea24b : Product
  Product_ff247 : Product
  Subtract_27c84 : Sum  Inputs=+-
  Blockout_d_iq_load_9_b592d : Outport
  wires:
  Constant_-376.991118430775_ad088/1 -> Product_c5042/1
  Product_ff247/1 -> Subtract_27c84/2
  State_id_load_9_95b0f/1 -> Product_c5042/2
  Add_7623c/1 -> Blockout_d_iq_load_9_b592d/1
  Constant_1024.44576485514_7c6f5/1 -> Product_ff247/1
  Product_ea24b/1 -> Add_7623c/2
  Product_c5042/1 -> Subtract_27c84/1
  State_iq_load_9_9ab5c/1 -> Product_ff247/2
  Constant_1663.3851206221_38dd2/1 -> Product_ea24b/1
  State_vq_bus_9_4829d/1 -> Product_ea24b/2
  Subtract_27c84/1 -> Add_7623c/1

== system case3/AC_1/d_vd_bus_1_block ==
  note: d_vd_bus_1 in case3
      | $37699111.8430775\,\mathrm{id}_{\mathrm{bus},1}+376.991118430775\,\mathrm{vq}_{\mathrm{bus},1}$
      | Automatically generated on 2025-10-31 19:01:54 .
  Alge_id_bus_1_f922c : Inport
  State_vq_bus_1_8af1f : Inport  Port=2
  Add_94278 : Sum
  Constant_376.991118430775_a751c : Constant  Value=376.991118430775
  Constant_37699111.8430775_6690f : Constant  Value=37699111.8430775
  Product_b434e : Product
  Product_da03a : Product
  Blockout_d_vd_bus_1_fbb6b : Outport
  wires:
  Constant_37699111.8430775_6690f/1 -> Product_da03a/1
  Product_b434e/1 -> Add_94278/2
  Alge_id_bus_1_f922c/1 -> Product_da03a/2
  Constant_376.991118430775_a751c/1 -> Product_b434e/1
  State_vq_bus_1_8af1f/1 -> Product_b434e/2
  Add_94278/1 -> Blockout_d_vd_bus_1_fbb6b/1
  Product_da03a/1 -> Add_94278/1

== system case3/AC_1/d_vd_bus_2_block ==
  note: d_vd_bus_2 in case3
      | $37699111.8430775\,\mathrm{id}_{\mathrm{bus},2}+376.991118430775\,\mathrm{vq}_{\mathrm{bus},2}$
      | Automatically generated on 2025-10-31 19:01:55 .
  Alge_id_bus_2_0b6c0 : Inport
  State_vq_bus_2_58237 : Inport  Port=2
  Add_4f813 : Sum
  Constant_376.991118430775_40a5e : Constant  Value=376.991118430775
  Constant_37699111.8430775_94d37 : Constant  Value=37699111.8430775
  Product_60d97 : Product
  Product_6eb18 : Product
  Blockout_d_vd_bus_2_67dfb : Outport
  wires:
  Constant_37699111.8430775_94d37/1 -> Product_60d97/1
  Product_6eb18/1 -> Add_4f813/2
  Alge_id_bus_2_0b6c0/1 -> Product_60d97/2
  Constant_376.991118430775_40a5e/1 -> Product_6eb18/1
  Product_60d97/1 -> Add_4f813/1
  State_vq_bus_2_58237/1 -> Product_6eb18/2
  Add_4f813/1 -> Blockout_d_vd_bus_2_67dfb/1

== system case3/AC_1/d_vd_bus_3_block ==
  note: d_vd_bus_3 in case3
      | $37699111.8430775\,\mathrm{id}_{\mathrm{bus},3}+376.991118430775\,\mathrm{vq}_{\mathrm{bus},3}$
      | Automatically generated on 2025-10-31 19:01:57 .
  Alge_id_bus_3_439ad : Inport
  State_vq_bus_3_ac889 : Inport  Port=2
  Add_ce32b : Sum
  Constant_376.991118430775_c1531 : Constant  Value=376.991118430775
  Constant_37699111.8430775_00b22 : Constant  Value=37699111.8430775
  Product_a79e8 : Product
  Product_fb7bd : Product
  Blockout_d_vd_bus_3_94704 : Outport
  wires:
  Constant_37699111.8430775_00b22/1 -> Product_a79e8/1
  Product_fb7bd/1 -> Add_ce32b/2
  Alge_id_bus_3_439ad/1 -> Product_a79e8/2
  Constant_376.991118430775_c1531/1 -> Product_fb7bd/1
  Product_a79e8/1 -> Add_ce32b/1
  State_vq_bus_3_ac889/1 -> Product_fb7bd/2
  Add_ce32b/1 -> Blockout_d_vd_bus_3_94704/1

== system case3/AC_1/d_vd_bus_4_block ==
  note: d_vd_bus_4 in case3
      | $2257.43184689087\,\mathrm{id}_{\mathrm{bus},4}+376.991118430775\,\mathrm{vq}_{\mathrm{bus},4}$
      | Automatically generated on 2025-10-31 19:01:58 .
  Alge_id_bus_4_7068c : Inport
  State_vq_bus_4_69940 : Inport  Port=2
  Add_357e5 : Sum
  Constant_2257.43184689087_214c1 : Constant  Value=2257.43184689087
  Constant_376.991118430775_f6230 : Constant  Value=376.991118430775
  Product_1e6ae : Product
  Product_fd7d5 : Product
  Blockout_d_vd_bus_4_12eb5 : Outport
  wires:
  Constant_2257.43184689087_214c1/1 -> Product_fd7d5/1
  Product_1e6ae/1 -> Add_357e5/2
  Alge_id_bus_4_7068c/1 -> Product_fd7d5/2
  Constant_376.991118430775_f6230/1 -> Product_1e6ae/1
  Product_fd7d5/1 -> Add_357e5/1
  State_vq_bus_4_69940/1 -> Product_1e6ae/2
  Add_357e5/1 -> Blockout_d_vd_bus_4_12eb5/1

== system case3/AC_1/d_vd_bus_5_block ==
  note: d_vd_bus_5 in case3
      | $1461.2058853906\,\mathrm{id}_{\mathrm{bus},5}+376.991118430775\,\mathrm{vq}_{\mathrm{bus},5}$
      | Automatically generated on 2025-10-31 19:02:00 .
  Alge_id_bus_5_5e52c : Inport
  State_vq_bus_5_467f2 : Inport  Port=2
  Add_9b0d0 : Sum
  Constant_1461.2058853906_ffc05 : Constant  Value=1461.2058853906
  Constant_376.991118430775_8c99d : Constant  Value=376.991118430775
  Product_146b3 : Product
  Product_8051b : Product
  Blockout_d_vd_bus_5_bd9e5 : Outport
  wires:
  Constant_1461.2058853906_ffc05/1 -> Product_146b3/1
  Product_8051b/1 -> Add_9b0d0/2
  Alge_id_bus_5_5e52c/1 -> Product_146b3/2
  Constant_376.991118430775_8c99d/1 -> Product_8051b/1
  Product_146b3/1 -> Add_9b0d0/1
  State_vq_bus_5_467f2/1 -> Product_8051b/2
  Add_9b0d0/1 -> Blockout_d_vd_bus_5_bd9e5/1

== system case3/AC_1/d_vd_bus_6_block ==
  note: d_vd_bus_6 in case3
      | $1329.77466818616\,\mathrm{id}_{\mathrm{bus},6}+376.991118430775\,\mathrm{vq}_{\mathrm{bus},6}$
      | Automatically generated on 2025-10-31 19:02:02 .
  Alge_id_bus_6_24922 : Inport
  State_vq_bus_6_63666 : Inport  Port=2
  Add_44085 : Sum
  Constant_1329.77466818616_10c16 : Constant  Value=1329.77466818616
  Constant_376.991118430775_9be69 : Constant  Value=376.991118430775
  Product_bc4a9 : Product
  Product_eb3f6 : Product
  Blockout_d_vd_bus_6_74d5d : Outport
  wires:
  Constant_1329.77466818616_10c16/1 -> Product_bc4a9/1
  Product_eb3f6/1 -> Add_44085/2
  Alge_id_bus_6_24922/1 -> Product_bc4a9/2
  Constant_376.991118430775_9be69/1 -> Product_eb3f6/1
  Product_bc4a9/1 -> Add_44085/1
  State_vq_bus_6_63666/1 -> Product_eb3f6/2
  Add_44085/1 -> Blockout_d_vd_bus_6_74d5d/1

== system case3/AC_1/d_vd_bus_7_block ==
  note: d_vd_bus_7 in case3
      | $2106.09563369148\,\mathrm{id}_{\mathrm{bus},7}+376.991118430775\,\mathrm{vq}_{\mathrm{bus},7}$
      | Automatically generated on 2025-10-31 19:02:03 .
  Alge_id_bus_7_2d419 : Inport
  State_vq_bus_7_8f28b : Inport  Port=2
  Add_0bc31 : Sum
  Constant_2106.09563369148_74a2b : Constant  Value=2106.09563369148
  Constant_376.991118430775_8fbcd : Constant  Value=376.991118430775
  Product_6cade : Product
  Product_7ba78 : Product
  Blockout_d_vd_bus_7_d7b36 : Outport
  wires:
  Constant_2106.09563369148_74a2b/1 -> Product_7ba78/1
  Product_6cade/1 -> Add_0bc31/2
  Alge_id_bus_7_2d419/1 -> Product_7ba78/2
  Constant_376.991118430775_8fbcd/1 -> Product_6cade/1
  Product_7ba78/1 -> Add_0bc31/1
  State_vq_bus_7_8f28b/1 -> Product_6cade/2
  Add_0bc31/1 -> Blockout_d_vd_bus_7_d7b36/1

== system case3/AC_1/d_vd_bus_8_block ==
  note: d_vd_bus_8 in case3
      | $1657.10381727813\,\mathrm{id}_{\mathrm{bus},8}+376.991118430775\,\mathrm{vq}_{\mathrm{bus},8}$
      | Automatically generated on 2025-10-31 19:02:05 .
  Alge_id_bus_8_ebbc1 : Inport
  State_vq_bus_8_8405d : Inport  Port=2
  Add_4792c : Sum
  Constant_1657.10381727813_167c7 : Constant  Value=1657.10381727813
  Constant_376.991118430775_16b7a : Constant  Value=376.991118430775
  Product_7bde4 : Product
  Product_de8eb : Product
  Blockout_d_vd_bus_8_98eda : Outport
  wires:
  Constant_1657.10381727813_167c7/1 -> Product_de8eb/1
  Product_7bde4/1 -> Add_4792c/2
  Alge_id_bus_8_ebbc1/1 -> Product_de8eb/2
  Constant_376.991118430775_16b7a/1 -> Product_7bde4/1
  Product_de8eb/1 -> Add_4792c/1
  State_vq_bus_8_8405d/1 -> Product_7bde4/2
  Add_4792c/1 -> Blockout_d_vd_bus_8_98eda/1

== system case3/AC_1/d_vd_bus_9_block ==
  note: d_vd_bus_9 in case3
      | $1564.27849971276\,\mathrm{id}_{\mathrm{bus},9}+376.991118430775\,\mathrm{vq}_{\mathrm{bus},9}$
      | Automatically generated on 2025-10-31 19:02:07 .
  Alge_id_bus_9_730d0 : Inport
  State_vq_bus_9_8a543 : Inport  Port=2
  Add_959d4 : Sum
  Constant_1564.27849971276_09e9a : Constant  Value=1564.27849971276
  Constant_376.991118430775_b49fd : Constant  Value=376.991118430775
  Product_3e959 : Product
  Product_4e792 : Product
  Blockout_d_vd_bus_9_9d4f1 : Outport
  wires:
  Constant_1564.27849971276_09e9a/1 -> Product_3e959/1
  Product_4e792/1 -> Add_959d4/2
  Alge_id_bus_9_730d0/1 -> Product_3e959/2
  Constant_376.991118430775_b49fd/1 -> Product_4e792/1
  Product_3e959/1 -> Add_959d4/1
  State_vq_bus_9_8a543/1 -> Product_4e792/2
  Add_959d4/1 -> Blockout_d_vd_bus_9_9d4f1/1

== system case3/AC_1/d_vq_bus_1_block ==
  note: d_vq_bus_1 in case3
      | $37699111.8430775\,\mathrm{iq}_{\mathrm{bus},1}-376.991118430775\,\mathrm{vd}_{\mathrm{bus},1}$
      | Automatically generated on 2025-10-31 19:01:54 .
  Alge_iq_bus_1_c886c : Inport
  State_vd_bus_1_0864e : Inport  Port=2
  Constant_376.991118430775_9ba15 : Constant  Value=376.991118430775
  Constant_37699111.8430775_24666 : Constant  Value=37699111.8430775
  Product_21965 : Product
  Product_23136 : Product
  Subtract_55d40 : Sum  Inputs=+-
  Blockout_d_vq_bus_1_6dae5 : Outport
  wires:
  Constant_37699111.8430775_24666/1 -> Product_21965/1
  Constant_376.991118430775_9ba15/1 -> Product_23136/1
  Alge_iq_bus_1_c886c/1 -> Product_21965/2
  State_vd_bus_1_0864e/1 -> Product_23136/2
  Product_21965/1 -> Subtract_55d40/1
  Product_23136/1 -> Subtract_55d40/2
  Subtract_55d40/1 -> Blockout_d_vq_bus_1_6dae5/1

== system case3/AC_1/d_vq_bus_2_block ==
  note: d_vq_bus_2 in case3
      | $37699111.8430775\,\mathrm{iq}_{\mathrm{bus},2}-376.991118430775\,\mathrm{vd}_{\mathrm{bus},2}$
      | Automatically generated on 2025-10-31 19:01:56 .
  Alge_iq_bus_2_2abe7 : Inport
  State_vd_bus_2_d00a9 : Inport  Port=2
  Constant_376.991118430775_5c7a3 : Constant  Value=376.991118430775
  Constant_37699111.8430775_7c047 : Constant  Value=37699111.8430775
  Product_19885 : Product
  Product_b52a9 : Product
  Subtract_90d3e : Sum  Inputs=+-
  Blockout_d_vq_bus_2_6ba06 : Outport
  wires:
  Constant_37699111.8430775_7c047/1 -> Product_b52a9/1
  Constant_376.991118430775_5c7a3/1 -> Product_19885/1
  Alge_iq_bus_2_2abe7/1 -> Product_b52a9/2
  State_vd_bus_2_d00a9/1 -> Product_19885/2
  Product_b52a9/1 -> Subtract_90d3e/1
  Product_19885/1 -> Subtract_90d3e/2
  Subtract_90d3e/1 -> Blockout_d_vq_bus_2_6ba06/1

== system case3/AC_1/d_vq_bus_3_block ==
  note: d_vq_bus_3 in case3
      | $37699111.8430775\,\mathrm{iq}_{\mathrm{bus},3}-376.991118430775\,\mathrm{vd}_{\mathrm{bus},3}$
      | Automatically generated on 2025-10-31 19:01:58 .
  Alge_iq_bus_3_adc3d : Inport
  State_vd_bus_3_4e169 : Inport  Port=2
  Constant_376.991118430775_66ff6 : Constant  Value=376.991118430775
  Constant_37699111.8430775_b97da : Constant  Value=37699111.8430775
  Product_2cfb2 : Product
  Product_98202 : Product
  Subtract_91831 : Sum  Inputs=+-
  Blockout_d_vq_bus_3_16c3e : Outport
  wires:
  Constant_37699111.8430775_b97da/1 -> Product_98202/1
  Constant_376.991118430775_66ff6/1 -> Product_2cfb2/1
  Alge_iq_bus_3_adc3d/1 -> Product_98202/2
  State_vd_bus_3_4e169/1 -> Product_2cfb2/2
  Product_98202/1 -> Subtract_91831/1
  Product_2cfb2/1 -> Subtract_91831/2
  Subtract_91831/1 -> Blockout_d_vq_bus_3_16c3e/1

== system case3/AC_1/d_vq_bus_4_block ==
  note: d_vq_bus_4 in case3
      | $2257.43184689087\,\mathrm{iq}_{\mathrm{bus},4}-376.991118430775\,\mathrm{vd}_{\mathrm{bus},4}$
      | Automatically generated on 2025-10-31 19:01:59 .
  Alge_iq_bus_4_f534f : Inport
  State_vd_bus_4_6453c : Inport  Port=2
  Constant_2257.43184689087_e3d6f : Constant  Value=2257.43184689087
  Constant_376.991118430775_742e1 : Constant  Value=376.991118430775
  Product_d2f22 : Product
  Product_e3270 : Product
  Subtract_9e228 : Sum  Inputs=+-
  Blockout_d_vq_bus_4_cec24 : Outport
  wires:
  Constant_2257.43184689087_e3d6f/1 -> Product_e3270/1
  Constant_376.991118430775_742e1/1 -> Product_d2f22/1
  Alge_iq_bus_4_f534f/1 -> Product_e3270/2
  State_vd_bus_4_6453c/1 -> Product_d2f22/2
  Product_e3270/1 -> Subtract_9e228/1
  Product_d2f22/1 -> Subtract_9e228/2
  Subtract_9e228/1 -> Blockout_d_vq_bus_4_cec24/1

== system case3/AC_1/d_vq_bus_5_block ==
  note: d_vq_bus_5 in case3
      | $1461.2058853906\,\mathrm{iq}_{\mathrm{bus},5}-376.991118430775\,\mathrm{vd}_{\mathrm{bus},5}$
      | Automatically generated on 2025-10-31 19:02:01 .
  Alge_iq_bus_5_f83f1 : Inport
  State_vd_bus_5_2a82f : Inport  Port=2
  Constant_1461.2058853906_5f1a6 : Constant  Value=1461.2058853906
  Constant_376.991118430775_be0a0 : Constant  Value=376.991118430775
  Product_9972f : Product
  Product_adadf : Product
  Subtract_9095a : Sum  Inputs=+-
  Blockout_d_vq_bus_5_ebd21 : Outport
  wires:
  Constant_1461.2058853906_5f1a6/1 -> Product_adadf/1
  Constant_376.991118430775_be0a0/1 -> Product_9972f/1
  Alge_iq_bus_5_f83f1/1 -> Product_adadf/2
  State_vd_bus_5_2a82f/1 -> Product_9972f/2
  Product_adadf/1 -> Subtract_9095a/1
  Product_9972f/1 -> Subtract_9095a/2
  Subtract_9095a/1 -> Blockout_d_vq_bus_5_ebd21/1

== system case3/AC_1/d_vq_bus_6_block ==
  note: d_vq_bus_6 in case3
      | $1329.77466818616\,\mathrm{iq}_{\mathrm{bus},6}-376.991118430775\,\mathrm{vd}_{\mathrm{bus},6}$
      | Automatically generated on 2025-10-31 19:02:03 .
  Alge_iq_bus_6_a58d3 : Inport
  State_vd_bus_6_2678b : Inport  Port=2
  Constant_1329.77466818616_73341 : Constant  Value=1329.77466818616
  Constant_376.991118430775_b52f8 : Constant  Value=376.991118430775
  Product_57b27 : Product
  Product_dee08 : Product
  Subtract_a1a11 : Sum  Inputs=+-
  Blockout_d_vq_bus_6_50300 : Outport
  wires:
  Constant_1329.77466818616_73341/1 -> Product_57b27/1
  Constant_376.991118430775_b52f8/1 -> Product_dee08/1
  Alge_iq_bus_6_a58d3/1 -> Product_57b27/2
  State_vd_bus_6_2678b/1 -> Product_dee08/2
  Product_57b27/1 -> Subtract_a1a11/1
  Product_dee08/1 -> Subtract_a1a11/2
  Subtract_a1a11/1 -> Blockout_d_vq_bus_6_50300/1
